simulink model "PDFuzzyAutopilot_2016a"  (R2020b)
settings: Solver=ode4  StartTime=0.0  StopTime=6000  FixedStep=1  RelTol=1e-3
libraries: fuzblock x1
settings Model: Creator=ngoan  LastModifiedBy=Long
settings OptimizationCC: LifeSpan=inf
settings DebuggingCC: UnconnectedInputMsg=none  UnconnectedOutputMsg=none  UnconnectedLineMsg=none  ArithmeticOperatorsInVariantConditions=warning
settings SFSimCC: CustomCodeUndefinedFunction=UseInterfaceOnly
settings CodeAppCC: StateflowObjectComments=on

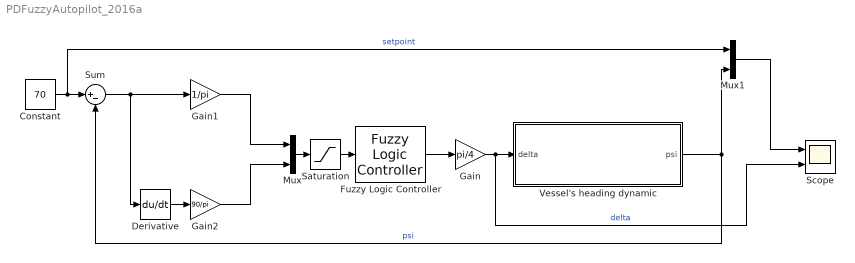
== system PDFuzzyAutopilot_2016a ==
  Constant : Constant  Value=70
  Derivative : Derivative
  Fuzzy Logic Controller : fuzblock/Fuzzy Logic  Controller  FIS='Autopilot_FuzzyController.fis'  OutputSampleNumber=101  DataType=double  FuzzifiedInputs=off  RuleFiringStrengths=off  RuleOutputs=off  AggregatedOutputs=off  SimulateUsing=Interpreted execution  OutOfRangeInputValueMessage=warning  NoRuleFiredMessage=warning  EmptyOutputFuzzySetMessage=warning
  Gain : Gain  Gain=pi/4
  Gain1 : Gain  Gain=1/pi
  Gain2 : Gain  Gain=90/pi
  Mux : Mux  Inputs=2
  Mux1 : Mux  Inputs=2
  Saturation : Saturate  UpperLimit=1  LowerLimit=-1
  Scope : Scope  NumInputPorts=2
  Sum : Sum  Inputs=|+-
  Vessel's heading dynamic : Subsystem
  wires:
  Gain/1 -> Scope/2, Vessel's heading dynamic/1(delta)  "delta"
  Fuzzy Logic Controller/1 -> Gain/1
  Gain1/1 -> Mux/1
  Gain2/1 -> Mux/2
  Mux/1 -> Saturation/1
  Vessel's heading dynamic/1(psi) -> Sum/2, Mux1/2  "psi"
  Sum/1 -> Derivative/1, Gain1/1
  Constant/1 -> Mux1/1, Sum/1  "setpoint"
  Derivative/1 -> Gain2/1
  Saturation/1 -> Fuzzy Logic Controller/1
  Mux1/1 -> Scope/1

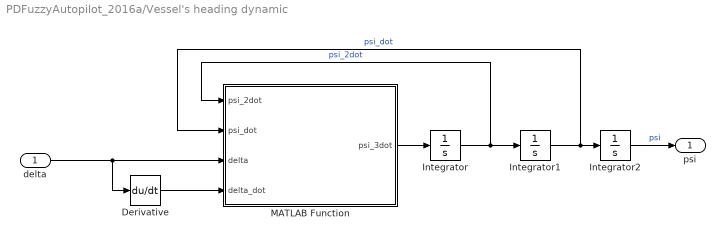
== system PDFuzzyAutopilot_2016a/Vessel's heading dynamic ==
  delta : Inport
  Derivative : Derivative
  Integrator : Integrator
  Integrator1 : Integrator
  Integrator2 : Integrator
  MATLAB Function : MATLAB Function  TreatAsAtomicUnit=on
  psi : Outport
  wires:
  delta/1 -> Derivative/1, MATLAB Function/3(delta)
  Integrator1/1 -> MATLAB Function/2(psi_dot), Integrator2/1  "psi_dot"
  MATLAB Function/1(psi_3dot) -> Integrator/1
  Derivative/1 -> MATLAB Function/4(delta_dot)
  Integrator/1 -> MATLAB Function/1(psi_2dot), Integrator1/1  "psi_2dot"
  Integrator2/1 -> psi/1  "psi"

== matlab function PDFuzzyAutopilot_2016a/Vessel's heading dynamic/MATLAB Function ==
  data: psi_2dot input; psi_3dot output; psi_dot input; delta input; delta_dot input
function psi_3dot = fcn(psi_2dot, psi_dot,delta,delta_dot)
l = 161 ; % vessel length
v = 5;  % vessel velocity
k0 = -3.86;
tau_10 = 5.66;
tau_20 = 0.38;
tau_30 = 0.89;
k = k0*v/l;
tau_1 = tau_10 *l/v;
tau_2 = tau_20 *l/v;
tau_3 = tau_30 *l/v;

psi_3dot = (k/(tau_1*tau_2))*(tau_3*delta_dot + delta)-(1/tau_1 +1/tau_2)*psi_2dot - (1/(tau_1*tau_2))*(psi_dot^3 +psi_dot);
